simulink model "hostSim"  (R2014b)
settings: Solver=ode45  StartTime=0.0  StopTime=10.0  RelTol=1e-3
undefined symbols (not defined in the file or in its folder): gcbh, rmidispblock
libraries: hostLogic x1
settings Model: DataDictionary=hostData.sldd  Creator=scastro  LastModifiedBy=scastro

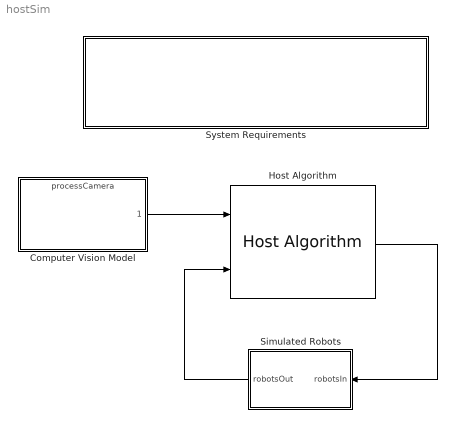
== system hostSim ==
  Computer Vision Model : ModelReference  ModelNameDialog=processCamera  SimulationMode=Normal  ModelReferenceVersion=1.2  CopyOfModelName=processCamera  DefaultDataLogging=on
  Host Algorithm : hostLogic/Host Algorithm
  Simulated Robots : Subsystem
  System Requirements : Subsystem  LoadFcn=rmidispblock('load',gcbh)  mask(System Requirements){id=SystemReq, title=System Requirements}
      mask prompts: title "Block Title"
      mask help: Lists the requirements for the current model.
      mask init:
      | id = 'SystemReq';
      | [w,h] = rmidispblock('display',gcbh);
      settings: CopyFcn=rmidispblock('create',gcbh)  DeleteFcn=rmidispblock('delete',gcbh)  ModelCloseFcn=rmidispblock('close',gcbh)  PreSaveFcn=rmidispblock('close',gcbh)  PostSaveFcn=rmidispblock('open',gcbh)  OpenFcn=rmidispblock('open',gcbh)  MoveFcn=rmidispblock('move',gcbh)
      mask Help: helpview(fullfile(docroot,'toolbox','slvnv','slvnv.map'),'systemrequirements')
      mask Display:
      | text(341/2,88-4,rmidispblock('title',gcbh),'horizontalAlignment','center','verticalAlignment','top')
      | text(w/2,h/2,'<No Requirements in System>','horizontalAlignment','center','verticalAlignment','top')
  wires:
  Computer Vision Model/1 -> Host Algorithm/1
  Host Algorithm/1 -> Simulated Robots/1(robotsIn)
  Simulated Robots/1(robotsOut) -> Host Algorithm/2

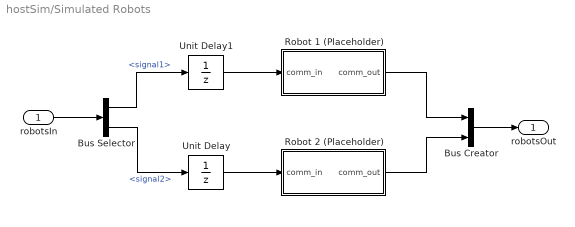
== system hostSim/Simulated Robots ==
  robotsIn : Inport
  Bus Creator : BusCreator  Inputs=2
  Bus Selector : BusSelector  OutputSignals=signal1,signal2
  Robot 1 (Placeholder) : Subsystem
  Robot 2 (Placeholder) : Subsystem
  Unit Delay : UnitDelay  SampleTime=-1
  Unit Delay1 : UnitDelay  SampleTime=-1
  robotsOut : Outport
  wires:
  robotsIn/1 -> Bus Selector/1
  Bus Selector/2 -> Unit Delay/1  "<signal2>"
  Robot 2 (Placeholder)/1(comm_out) -> Bus Creator/2
  Bus Creator/1 -> robotsOut/1
  Robot 1 (Placeholder)/1(comm_out) -> Bus Creator/1
  Unit Delay/1 -> Robot 2 (Placeholder)/1(comm_in)
  Unit Delay1/1 -> Robot 1 (Placeholder)/1(comm_in)
  Bus Selector/1 -> Unit Delay1/1  "<signal1>"

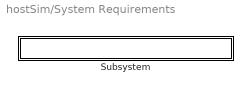
== system hostSim/System Requirements ==
  Subsystem : Subsystem  mask{label=0, index=1}
      mask init:
      | label = rmidispblock('label',index);
      settings: OpenFcn=rmidispblock('openReq',gcbh);
      mask Display: text(0,0,label,'horizontalAlignment','left','verticalAlignment','bottom')

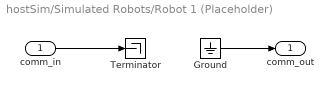
== system hostSim/Simulated Robots/Robot 1 (Placeholder) ==
  comm_in : Inport
  Ground : Ground
  Terminator : Terminator
  comm_out : Outport
  wires:
  Ground/1 -> comm_out/1
  comm_in/1 -> Terminator/1

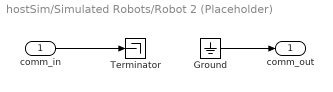
== system hostSim/Simulated Robots/Robot 2 (Placeholder) ==
  comm_in : Inport
  Ground : Ground
  Terminator : Terminator
  comm_out : Outport
  wires:
  comm_in/1 -> Terminator/1
  Ground/1 -> comm_out/1

== system hostSim/System Requirements/Subsystem ==
